simulink model "Controller"  (R2020b)
settings: Solver=ode1  StartTime=0.0  StopTime=10  FixedStep=1e-3  RelTol=1e-3
values from neighbouring files (symbols this model uses):
  bin = [0.818045624381 0.102878023448 0.737296135799 0.38218842541 0.977505309906 0.149360203196 0.641439600547 0.443497484934 0.68042192531 0.859879825833 -0.31868948267 0.255207188653 ... (20 elements, 20x1)]    [052data.mat]
  Win = [0.811661315568 0.781547366352 0.146098503423 0.266102211582 0.397284814094 0.516628753495 0.0862525926602 0.103414091455 0.506698658208 0.269175608562 0.0151134208658 0.873047701594 ... (40 elements, 20x2)]    [052data.mat]
  Wout = [0.610759087178 0.366179666335 -0.0584030572952 0.209075859993 0.584389586359 0.349871470562 -0.204405272266 -0.116182445469 0.0642557952818 -0.132902026264 0.805831183297 -0.399691016291 ... (20 elements, 1x20)]    [052data.mat]
libraries: pid_lib x1
settings Model: Creator=yarat  LastModifiedBy=yarat

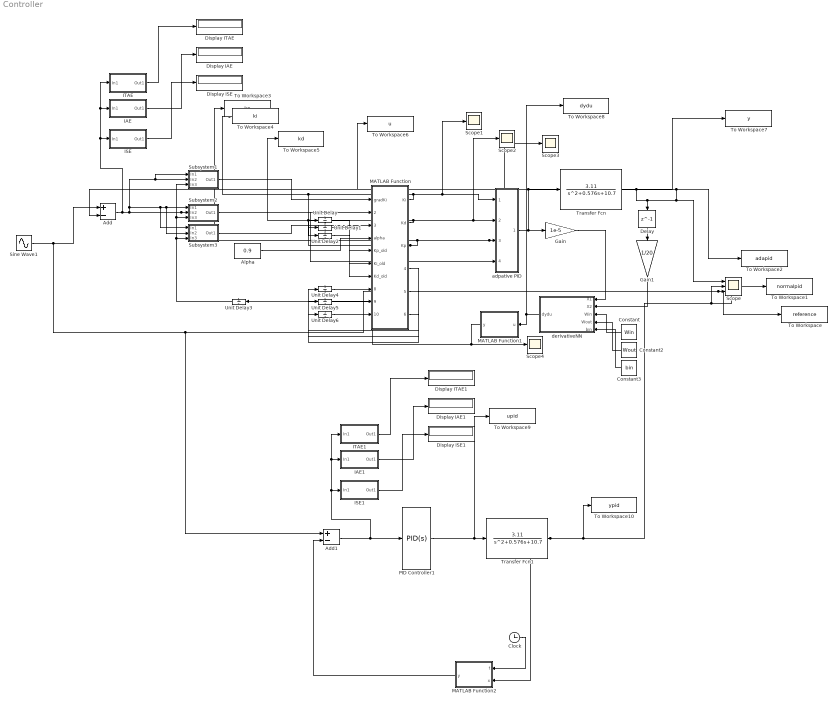
== system Controller ==
  Add : Sum  Inputs=+-
  Add1 : Sum  Inputs=+-
  Alpha : Constant  Value=0.9
  Clock : Clock
  Constant : Constant  Value=Win
  Constant2 : Constant  Value=Wout
  Constant3 : Constant  Value=bin
  Delay : Delay  DelayLength=1  SampleTime=1e-3
  Display IAE : Display
  Display IAE1 : Display
  Display ISE : Display
  Display ISE1 : Display
  Display ITAE : Display
  Display ITAE1 : Display
  Gain : Gain  Gain=1e-5
  Gain1 : Gain  Gain=1/20
  IAE : Subsystem
      mask help:
      | IAE performacne index
      |
      | output = int |input| dt
      mask Display:
      | disp('IAE')
      | port_label('input',1,'e')
      | port_label('output',1,'iae')
  IAE1 : Subsystem
      mask help:
      | IAE performacne index
      |
      | output = int |input| dt
      mask Display:
      | disp('IAE')
      | port_label('input',1,'e')
      | port_label('output',1,'iae')
  ISE : Subsystem
      mask help:
      | ISE performance index
      |
      | output = int (input)^2 dt
      mask Display:
      | disp('ISE')
      | port_label('input',1,'e')
      | port_label('output',1,'ise')
  ISE1 : Subsystem
      mask help:
      | ISE performance index
      |
      | output = int (input)^2 dt
      mask Display:
      | disp('ISE')
      | port_label('input',1,'e')
      | port_label('output',1,'ise')
  ITAE : Subsystem
      mask help:
      | ITAE performance index
      |
      | output = int t|input| dt
      mask Display:
      | disp('ITAE')
      | port_label('input',1,'e')
      | port_label('output',1,'itae')
  ITAE1 : Subsystem
      mask help:
      | ITAE performance index
      |
      | output = int t|input| dt
      mask Display:
      | disp('ITAE')
      | port_label('input',1,'e')
      | port_label('output',1,'itae')
  MATLAB Function : MATLAB Function  TreatAsAtomicUnit=on
  MATLAB Function1 : MATLAB Function  TreatAsAtomicUnit=on
  MATLAB Function2 : MATLAB Function  TreatAsAtomicUnit=on
  PID Controller1 : pid_lib/PID Controller  Controller=PID  Form=Parallel  TimeDomain=Continuous-time  UseExternalTs=off  SampleTime=-1  IntegratorMethod=Forward Euler  FilterMethod=Forward Euler  ControllerParametersSource=internal  P=17.9012745706573  I=22.4780602564623  D=3.11340256685474  UseFilter=on  N=43.6837145784617  TunerSelectOption=Transfer Function Based (PID Tuner App)  InitialConditionSource=internal  InitialConditionForIntegrator=0  InitialConditionForFilter=0  DifferentiatorICPrevScaledInput=0  ExternalReset=none  TrackingMode=off  Kt=1  LimitOutput=off  SatLimitsSource=internal  UpperSaturationLimit=inf  LowerSaturationLimit=-inf  LinearizeAsGain=on  AntiWindupMode=none  Kb=1  POutMin=[]  POutMax=[]  IOutMin=[]  IOutMax=[]  DOutMin=[]  DOutMax=[]  NOutMin=[]  NOutMax=[]  SumOutMin=[]  SumOutMax=[]  SaturationOutMin=[]  SaturationOutMax=[]  PParamMin=[]  PParamMax=[]  IParamMin=[]  IParamMax=[]  DParamMin=[]  DParamMax=[]  NParamMin=[]  NParamMax=[]  KbParamMin=[]  KbParamMax=[]  KtParamMin=[]  KtParamMax=[]  KbOutMin=[]  KbOutMax=[]  KtOutMin=[]  KtOutMax=[]  IntegratorOutMin=[]  IntegratorOutMax=[]  FilterOutMin=[]  FilterOutMax=[]  SumI1OutMin=[]  SumI1OutMax=[]  SumI2OutMin=[]  SumI2OutMax=[]  SumI3OutMin=[]  SumI3OutMax=[]  SumI4OutMin=[]  SumI4OutMax=[]  SumDOutMin=[]  SumDOutMax=[]  DifferentiatorOutMin=[]  DifferentiatorOutMax=[]  FilterDiffOutCoefMin=[]  FilterDiffOutCoefMax=[]  ReciprocalOutMin=[]  ReciprocalOutMax=[]  SumDenOutMin=[]  SumDenOutMax=[]  SumNumOutMin=[]  SumNumOutMax=[]  DivideOutMin=[]  DivideOutMax=[]  UdiffTsProdOutMin=[]  UdiffTsProdOutMax=[]  NTsProdOutMin=[]  NTsProdOutMax=[]  UintegralTsProdOutMin=[]  UintegralTsProdOutMax=[]  UngainTsProdOutMin=[]  UngainTsProdOutMax=[]  IntegratorContinuousStateAttributes=''  IntegratorStateMustResolveToSignalObject=off  IntegratorRTWStateStorageClass=Auto  FilterContinuousStateAttributes=''  FilterStateMustResolveToSignalObject=off  FilterRTWStateStorageClass=Auto  ParallelPVariant=InternalParameters  IdealPVariant=Disabled  IVariant=InternalParameters  DVariant=InternalParameters  IntegratorVariant=Continuous  SatVariant=Disabled  AWVariant=Passthrough  PCopyVariant=Disabled  TRVariant=Disabled  FdbkBlocksVariant=Forward  IdealPFdbkVariant=Disabled  SatFdbkVariant=Disabled  DerivativeFilterVariant=ContFilter  NVariant=InternalParameters  NCopyVariant=Disabled  FilterICVariant=InternalICsFilter  IntegratorICVariant=InternalICs  ExternalResetVariant=Disabled  TRSumVariant=Passthrough  SumFdbkVariant=Disabled  SumVariant=Sum_PID  TsampFilterVariant=InternalTs  TsampNgainVariant=Passthrough  TsampIntegralVariant=Passthrough  ExternalSaturationOutDataTypeStr=Inherit: Same as second input
  Scope : Scope  NumInputPorts=3
  Scope{1..4} (4 alike) : Scope
  Sine Wave1 : Sin  Amplitude=0.2  Frequency=2*pi  SampleTime=0
  Subsystem1 : Subsystem
  Subsystem2 : Subsystem
  Subsystem3 : Subsystem
  To Workspace : ToWorkspace  VariableName=reference  SampleTime=-1
  To Workspace1 : ToWorkspace  VariableName=normalpid  SampleTime=-1
  To Workspace10 : ToWorkspace  VariableName=ypid  SampleTime=-1
  To Workspace2 : ToWorkspace  VariableName=adapid  SampleTime=-1
  To Workspace3 : ToWorkspace  VariableName=kp  SampleTime=-1
  To Workspace4 : ToWorkspace  VariableName=ki  SampleTime=-1
  To Workspace5 : ToWorkspace  VariableName=kd  SampleTime=-1
  To Workspace6 : ToWorkspace  VariableName=u  SampleTime=-1
  To Workspace7 : ToWorkspace  VariableName=y  SampleTime=-1
  To Workspace8 : ToWorkspace  VariableName=dydu  SampleTime=-1
  To Workspace9 : ToWorkspace  VariableName=upid  SampleTime=-1
  Transfer Fcn : TransferFcn  Numerator=[3.11]  Denominator=[1 0.576 10.7]
  Transfer Fcn1 : TransferFcn  Numerator=[3.11]  Denominator=[1 0.576 10.7]
  Unit Delay : UnitDelay  InitialCondition=29  SampleTime=1e-3  HasFrameUpgradeWarning=on
  Unit Delay1 : UnitDelay  InitialCondition=34  SampleTime=1e-3  HasFrameUpgradeWarning=on
  Unit Delay2 : UnitDelay  InitialCondition=4  SampleTime=1e-3  HasFrameUpgradeWarning=on
  Unit Delay{3..6} (4 alike) : UnitDelay  SampleTime=1e-3  HasFrameUpgradeWarning=on
  adpative PID : Subsystem
  derivativeNN : MATLAB Function  TreatAsAtomicUnit=on
  wires:
  adpative PID/1(Out1) -> Gain/1, Transfer Fcn/1, To Workspace6/1
  Sine Wave1/1 -> Add/1, Add1/1, To Workspace/1, Scope/3
  Add/1 -> ITAE/1(In1), IAE/1(In1), ISE/1(In1), Subsystem2/2(In2), adpative PID/4(In4), Subsystem1/2(In2), Subsystem1/1(In1), Subsystem3/1(In1), Subsystem3/2(In2), Subsystem2/1(In1)
  derivativeNN/1(dydu) -> MATLAB Function1/1(u), To Workspace8/1
  MATLAB Function/1(Ki) -> To Workspace4/1, Unit Delay1/1, adpative PID/1(In1), Scope1/1
  MATLAB Function/2(Kd) -> To Workspace5/1, Unit Delay2/1, adpative PID/2(In3), Scope2/1
  MATLAB Function/3(Kp) -> Unit Delay/1, Scope3/1, adpative PID/3(In2), To Workspace3/1
  Subsystem2/1(Out1) -> MATLAB Function/2(gradKd)
  Subsystem3/1(Out1) -> MATLAB Function/3(gradKp)
  Alpha/1 -> MATLAB Function/4(alpha)
  Subsystem1/1(Out1) -> MATLAB Function/1(gradKi)
  Unit Delay/1 -> MATLAB Function/5(Kp_old)
  Unit Delay1/1 -> MATLAB Function/6(Ki_old)
  Unit Delay2/1 -> MATLAB Function/7(Kd_old)
  Unit Delay3/1 -> Subsystem3/3(In3), Subsystem2/3(In3), Subsystem1/3(In3)
  Unit Delay4/1 -> MATLAB Function/8("gradKp_old ")
  Unit Delay5/1 -> MATLAB Function/9("gradKi_old ")
  Unit Delay6/1 -> MATLAB Function/10("gradKd_old ")
  MATLAB Function/4(gradKp_old) -> Unit Delay4/1
  MATLAB Function/5(gradKi_old) -> Unit Delay5/1
  MATLAB Function/6(gradKd_old) -> Unit Delay6/1
  Constant/1 -> derivativeNN/3(Win)
  Constant2/1 -> derivativeNN/4(Wout)
  Constant3/1 -> derivativeNN/5(bin)
  Gain/1 -> derivativeNN/1(X1)
  Delay/1 -> Gain1/1
  MATLAB Function1/1(y) -> Scope4/1, Unit Delay3/1
  Transfer Fcn1/1 -> To Workspace10/1, To Workspace1/1, Scope/2, MATLAB Function2/2(x)
  MATLAB Function2/1(y) -> Add1/2
  Clock/1 -> MATLAB Function2/1(t)
  Gain1/1 -> derivativeNN/2(X2)
  PID Controller1/1 -> To Workspace9/1, Transfer Fcn1/1
  Transfer Fcn/1 -> To Workspace7/1, Scope/1, To Workspace2/1, Add/2, Delay/1
  ITAE/1(Out1) -> Display ITAE/1
  ISE/1(Out1) -> Display ISE/1
  IAE/1(Out1) -> Display IAE/1
  IAE1/1(Out1) -> Display IAE1/1
  Add1/1 -> ITAE1/1(In1), IAE1/1(In1), ISE1/1(In1), PID Controller1/1
  ITAE1/1(Out1) -> Display ITAE1/1
  ISE1/1(Out1) -> Display ISE1/1

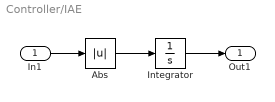
== system Controller/IAE ==
  In1 : Inport
  Abs : Abs
  Integrator : Integrator
  Out1 : Outport
  wires:
  In1/1 -> Abs/1
  Integrator/1 -> Out1/1
  Abs/1 -> Integrator/1

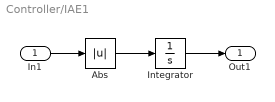
== system Controller/IAE1 ==
  In1 : Inport
  Abs : Abs
  Integrator : Integrator
  Out1 : Outport
  wires:
  In1/1 -> Abs/1
  Integrator/1 -> Out1/1
  Abs/1 -> Integrator/1

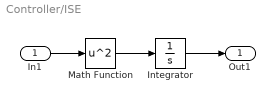
== system Controller/ISE ==
  In1 : Inport
  Integrator : Integrator
  Math Function : Math  Operator=square  SignedPower=on  SaturateOnIntegerOverflow=on
  Out1 : Outport
  wires:
  Math Function/1 -> Integrator/1
  Integrator/1 -> Out1/1
  In1/1 -> Math Function/1

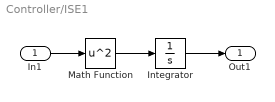
== system Controller/ISE1 ==
  In1 : Inport
  Integrator : Integrator
  Math Function : Math  Operator=square  SignedPower=on  SaturateOnIntegerOverflow=on
  Out1 : Outport
  wires:
  Math Function/1 -> Integrator/1
  Integrator/1 -> Out1/1
  In1/1 -> Math Function/1

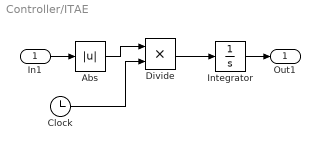
== system Controller/ITAE ==
  In1 : Inport
  Abs : Abs
  Clock : Clock
  Divide : Product  Inputs=**
  Integrator : Integrator
  Out1 : Outport
  wires:
  Integrator/1 -> Out1/1
  In1/1 -> Abs/1
  Divide/1 -> Integrator/1
  Abs/1 -> Divide/1
  Clock/1 -> Divide/2

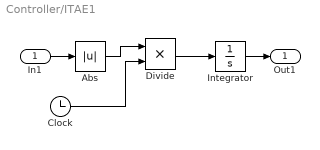
== system Controller/ITAE1 ==
  In1 : Inport
  Abs : Abs
  Clock : Clock
  Divide : Product  Inputs=**
  Integrator : Integrator
  Out1 : Outport
  wires:
  Integrator/1 -> Out1/1
  In1/1 -> Abs/1
  Divide/1 -> Integrator/1
  Abs/1 -> Divide/1
  Clock/1 -> Divide/2

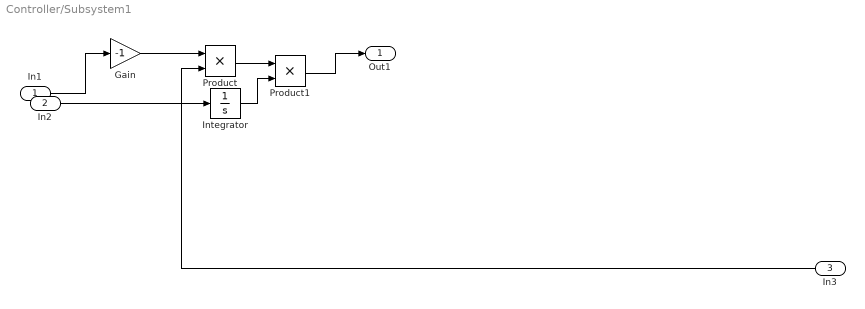
== system Controller/Subsystem1 ==
  In1 : Inport
  In2 : Inport  Port=2
  In3 : Inport  Port=3
  Gain : Gain  Gain=-1
  Integrator : Integrator
  Product : Product
  Product1 : Product
  Out1 : Outport
  wires:
  Integrator/1 -> Product1/2
  Gain/1 -> Product/1
  Product1/1 -> Out1/1
  Product/1 -> Product1/1
  In2/1 -> Integrator/1
  In3/1 -> Product/2
  In1/1 -> Gain/1

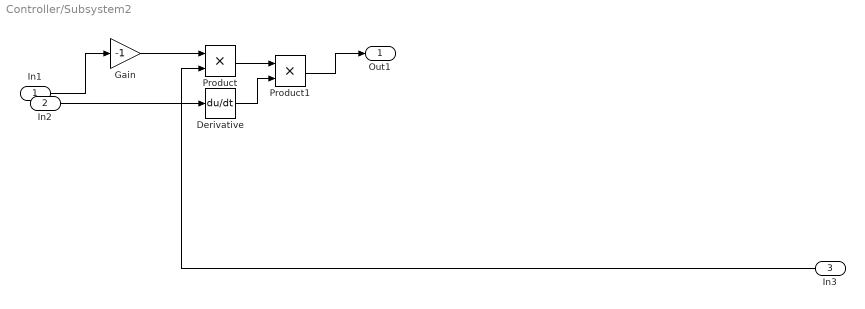
== system Controller/Subsystem2 ==
  In1 : Inport
  In2 : Inport  Port=2
  In3 : Inport  Port=3
  Derivative : Derivative
  Gain : Gain  Gain=-1
  Product : Product
  Product1 : Product
  Out1 : Outport
  wires:
  In1/1 -> Gain/1
  In3/1 -> Product/2
  In2/1 -> Derivative/1
  Product/1 -> Product1/1
  Product1/1 -> Out1/1
  Gain/1 -> Product/1
  Derivative/1 -> Product1/2

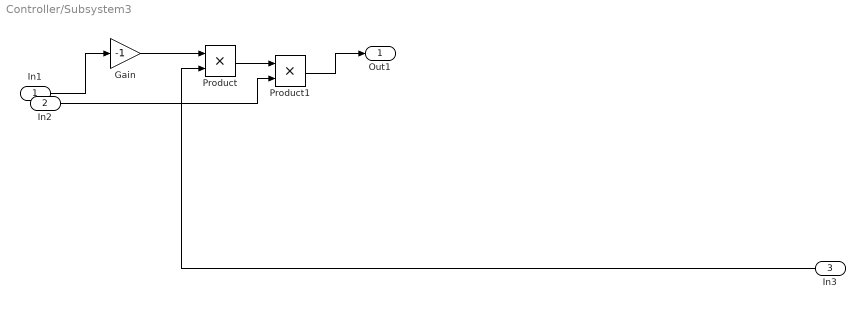
== system Controller/Subsystem3 ==
  In1 : Inport
  In2 : Inport  Port=2
  In3 : Inport  Port=3
  Gain : Gain  Gain=-1
  Product : Product
  Product1 : Product
  Out1 : Outport
  wires:
  In2/1 -> Product1/2
  Gain/1 -> Product/1
  Product1/1 -> Out1/1
  Product/1 -> Product1/1
  In3/1 -> Product/2
  In1/1 -> Gain/1

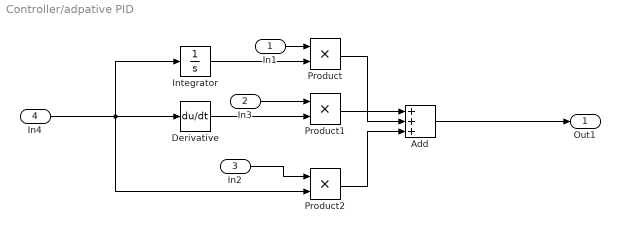
== system Controller/adpative PID ==
  In1 : Inport
  In3 : Inport  Port=2
  In2 : Inport  Port=3
  In4 : Inport  Port=4
  Add : Sum  Inputs=+++
  Derivative : Derivative
  Integrator : Integrator
  Product : Product
  Product1 : Product
  Product2 : Product
  Out1 : Outport
  wires:
  Integrator/1 -> Product/2
  In2/1 -> Product2/1
  In4/1 -> Product2/2, Derivative/1, Integrator/1
  Product/1 -> Add/2
  Product1/1 -> Add/1
  Product2/1 -> Add/3
  Derivative/1 -> Product1/2
  In3/1 -> Product1/1
  In1/1 -> Product/1
  Add/1 -> Out1/1

== matlab function Controller/derivativeNN ==
  data: X1 input size=[1,1]; X2 input size=[1,1]; dydu output size=[1,1]; Win input size=[20,2]; Wout input size=[1,20]; bin input size=[20,1]

function dydu  = ffnetforcast(X1,X2, Win, Wout, bin)
X = [X1;X2];
netin = Win*X + bin;
dydu_pre = Win'*(Wout'.*hprime(netin));
dydu = dydu_pre(1,1);
function y = hprime(x)
    y = (1-tanh(x).^2);
end
end

== matlab function Controller/MATLAB Function ==
  data: gradKi input; Ki output; gradKd input; gradKp input; Kd output; Kp output; alpha input; Kp_old input; Ki_old input; Kd_old input; gradKp_old input; gradKi_old input; gradKd_old input; gradKp_old output; gradKi_old output; gradKd_old output
function [Ki,Kd,Kp,gradKp_old,gradKi_old,gradKd_old] = fcn(gradKi,gradKd,gradKp, alpha, Kp_old, Ki_old, Kd_old,gradKp_old,gradKi_old,gradKd_old)



% v = beta*(oldGrad) + (1-beta)*grad;
% oldGrad = v;
% param = param - alpha*v;
beta = 0.8;
Vkp = beta*gradKp_old + (1-beta)*gradKp;
Vki = beta*gradKi_old + (1-beta)*gradKi;
Vkd = beta*gradKd_old + (1-beta)*gradKd;

Kp = Kp_old - alpha*Vkp;
Ki = Ki_old - alpha*Vki;
Kd = Kd_old - alpha*Vkd;

gradKp_old = Vkp;
gradKi_old = Vki;
gradKd_old = Vkd;


end

== matlab function Controller/MATLAB Function1 ==
  data: u input; y output
function y = fcn(u)
if u == 0
    y = 0.0001;
else
y = u;
end

== matlab function Controller/MATLAB Function2 ==
  data: t input; y output; x input
function y = fcn(t,x)
if t>50
    y = x +0.5;
else
    y = x +0;
end
